simulink model "Deepanshu_GWO"  (R2021a)
settings: Solver=VariableStepAuto  StartTime=0.0  StopTime=20  FixedStep=1e-6  RelTol=1e-3
InitFcn:
  | global vv;
libraries: spsSeriesRLCBranchLib x9, spsDiodeLib x4, spsPVArrayLib x3, spsVoltageMeasurementLib x3, spsCurrentMeasurementLib x2, spsDCVoltageSourceLib x1, spsMosfetLib x1, eePwmGenerator x1, spspowerguiLib x1
settings Model: Creator=dfcpstage17  LastModifiedBy=sanr14
settings DebuggingCC: UnconnectedInputMsg=none  UnconnectedOutputMsg=none  UnconnectedLineMsg=none
settings RTWCC: DLArmComputeVersion=20.02.1

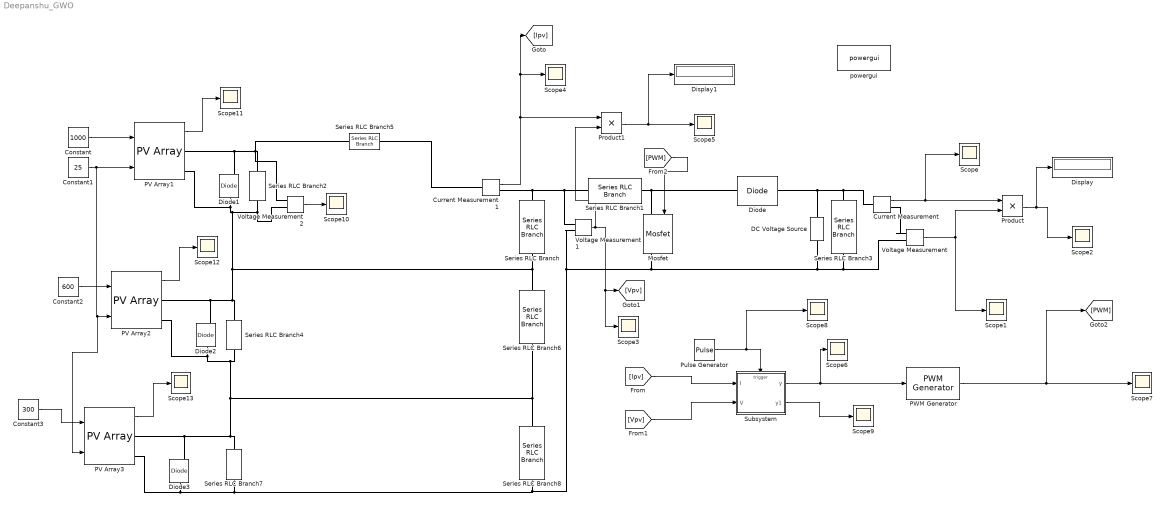
== system Deepanshu_GWO ==
  Constant : Constant  Value=1000
  Constant1 : Constant  Value=25
  Constant2 : Constant  Value=600
  Constant3 : Constant  Value=300
  Current Measurement : spsCurrentMeasurementLib/Current Measurement  PhasorSimulation=off  OutputType=Complex  PSBequivalent=0
  Current Measurement1 : spsCurrentMeasurementLib/Current Measurement  PhasorSimulation=off  OutputType=Complex  PSBequivalent=0
  DC Voltage Source : spsDCVoltageSourceLib/DC Voltage Source  Amplitude=80  Measurements=None
  Diode : spsDiodeLib/Diode  Ron=0.001  Lon=0  Vf=0.8  IC=0  UseSnubber=0  Rs=500  Cs=250e-9  Measurements=off
  Diode1 : spsDiodeLib/Diode  Ron=0.001  Lon=0  Vf=0.8  IC=0  UseSnubber=0  Rs=inf  Cs=inf  Measurements=on
  Diode2 : spsDiodeLib/Diode  Ron=0.001  Lon=0  Vf=0.8  IC=0  UseSnubber=0  Rs=inf  Cs=inf  Measurements=on
  Diode3 : spsDiodeLib/Diode  Ron=0.001  Lon=0  Vf=0.8  IC=0  UseSnubber=0  Rs=inf  Cs=inf  Measurements=on
  Display : Display
  Display1 : Display
  Mosfet : spsMosfetLib/Mosfet  Ron=0.1  Lon=0  Rd=0.01  Vfd=0  IC=0  Rs=1e5  Cs=inf  Measurements=on
  PV Array1 : spsPVArrayLib/PV Array  Npar=1  Nser=1  PlotType=array @ 1000 W/m2 & specified temperatures  S_vec="[ 1000  500  100 ]"  Temp_C_vec="[ 45 25  ]"  ModuleName=User-defined  PlotWhenSelected=off  Pm=86.996  Ncell=36  Voc=21  Isc=5.17  Vm=18.2  Im=4.78  beta_Voc_pc=-0.3616  alpha_Isc_pc=0.041509  beta_Voc=-0.075936  alpha_Isc=0.002146  IL=5.1832  I0=1.7804e-10  nI=0.94398  Rsh=97.5456  Rs=0.017583  RobustModel=off  RobustCellTemperature=313.3991  BAL=on  Tc=1e-6  Tfilter=5e-5
  PV Array2 : spsPVArrayLib/PV Array  Npar=1  Nser=1  PlotType=array @ 1000 W/m2 & specified temperatures  S_vec="[ 1000  500  100 ]"  Temp_C_vec="[ 45 25  ]"  ModuleName=User-defined  PlotWhenSelected=off  Pm=86.996  Ncell=36  Voc=21  Isc=5.17  Vm=18.2  Im=4.78  beta_Voc_pc=-0.3616  alpha_Isc_pc=0.041509  beta_Voc=-0.075936  alpha_Isc=0.002146  IL=5.1832  I0=1.7804e-10  nI=0.94398  Rsh=97.5456  Rs=0.017583  RobustModel=off  RobustCellTemperature=313.3991  BAL=on  Tc=1e-6  Tfilter=5e-5
  PV Array3 : spsPVArrayLib/PV Array  Npar=1  Nser=1  PlotType=array @ 1000 W/m2 & specified temperatures  S_vec="[ 1000  500  100 ]"  Temp_C_vec="[ 45 25  ]"  ModuleName=User-defined  PlotWhenSelected=off  Pm=86.996  Ncell=36  Voc=21  Isc=5.17  Vm=18.2  Im=4.78  beta_Voc_pc=-0.3616  alpha_Isc_pc=0.041509  beta_Voc=-0.075936  alpha_Isc=0.002146  IL=5.1832  I0=1.7804e-10  nI=0.94398  Rsh=97.5456  Rs=0.017583  RobustModel=off  RobustCellTemperature=313.3991  BAL=on  Tc=1e-6  Tfilter=5e-5
  PWM Generator : eePwmGenerator/PWM Generator  CarrCount=Up  Tper=0.0001  Ts=5e-6
  Product : Product
  Product1 : Product
  Pulse Generator : DiscretePulseGenerator  PulseType=Time based  Period=0.2  PulseWidth=30  PhaseDelay=1e-6
  Scope{,1..13} (14 alike) : Scope
  Series RLC Branch : spsSeriesRLCBranchLib/Series RLC Branch  LConnTagsString=__new0  RConnTagsString=__new0  BranchType=C  Resistance=1  Inductance=1e-3  SetiL0=off  InitialCurrent=0  Capacitance=1000e-6  Setx0=off  InitialVoltage=0  Measurements=None
  Series RLC Branch1 : spsSeriesRLCBranchLib/Series RLC Branch  LConnTagsString=__new0  RConnTagsString=__new0  BranchType=L  Resistance=1  Inductance=1e-3  SetiL0=off  InitialCurrent=0  Capacitance=1e-6  Setx0=off  InitialVoltage=0  Measurements=None
  Series RLC Branch{2..4,7} (4 alike) : spsSeriesRLCBranchLib/Series RLC Branch  LConnTagsString=__new0  RConnTagsString=__new0  BranchType=R  Resistance=100  Inductance=1e-3  SetiL0=off  InitialCurrent=0  Capacitance=1e-6  Setx0=off  InitialVoltage=0  Measurements=None
  Series RLC Branch5 : spsSeriesRLCBranchLib/Series RLC Branch  LConnTagsString=__new0  RConnTagsString=__new0  BranchType=R  Resistance=0.01  Inductance=1e-3  SetiL0=off  InitialCurrent=0  Capacitance=1e-6  Setx0=off  InitialVoltage=0  Measurements=None
  Series RLC Branch6 : spsSeriesRLCBranchLib/Series RLC Branch  LConnTagsString=__new0  RConnTagsString=__new0  BranchType=C  Resistance=1  Inductance=1e-3  SetiL0=off  InitialCurrent=0  Capacitance=1000e-6  Setx0=off  InitialVoltage=0  Measurements=None
  Series RLC Branch8 : spsSeriesRLCBranchLib/Series RLC Branch  LConnTagsString=__new0  RConnTagsString=__new0  BranchType=C  Resistance=1  Inductance=1e-3  SetiL0=off  InitialCurrent=0  Capacitance=1000e-6  Setx0=off  InitialVoltage=0  Measurements=None
  Subsystem : Subsystem
  Voltage Measurement : spsVoltageMeasurementLib/Voltage Measurement  PhasorSimulation=off  OutputType=Complex  PSBequivalent=0
  Voltage Measurement1 : spsVoltageMeasurementLib/Voltage Measurement  PhasorSimulation=off  OutputType=Complex  PSBequivalent=0
  Voltage Measurement2 : spsVoltageMeasurementLib/Voltage Measurement  PhasorSimulation=off  OutputType=Complex  PSBequivalent=0
  powergui : spspowerguiLib/powergui  Priority=1  SimulationMode=Discrete  SampleTime=1e-6  frequency=60  Iterations=50  frequencyindice=0  Pbase=100e6  ErrMax=1e-4  UnitsV=kV  UnitsW=MW  buscounter=0  FunctionMessages=off  echomessages=off  EnableUseOfTLC=off  CurrentSourceSwitches=off  DisableSnubberDevices=off  DisableRonSwitches=off  DisableVfSwitches=off  DisplayEquations=off  AutomaticDiscreteSolvers=off  SolverType=Tustin/Backward Euler (TBE)  Interpol=off  ExternalGateDelay=off  methode=off  Ts=100  x0status=blocks  SPID=on  SwTol=0  HookPort=off  NonlinearTolerance=1e-4  nMaxIteration=100  ContinueOnMaxIteration=off  RestoreLinks=warning  ResistiveCurrentMeasurement=off  Frange=[0:2:500]  Ylog=off  Xlog=on  ShowGrid=off  save=off  variable=ZData  structure=0  ZoomFFT=off  StartTime=0.0  cycles=1  DisplayStyle=1  fundamental=60  FreqAxis=off  MaxFrequency=1000  frequencyindicesteady=1  RmsSteady=1  display=off
  wires:
  Current Measurement/1 -> Scope/1, Product/1
  Voltage Measurement/1 -> Product/2, Scope1/1
  Product/1 -> Display/1, Scope2/1
  Voltage Measurement1/1 -> Product1/2, [Vpv], Scope3/1
  Current Measurement1/1 -> Product1/1, [Ipv], Scope4/1
  Product1/1 -> Display1/1, Scope5/1
  [Ipv] -> Subsystem/1(I)
  [Vpv] -> Subsystem/2(V)
  Pulse Generator/1 -> Scope8/1, Subsystem/Trigger
  PWM Generator/1 -> Scope7/1, [PWM]
  [PWM] -> Mosfet/1
  Subsystem/1(y) -> Scope6/1, PWM Generator/1
  Constant/1 -> PV Array1/1
  Constant1/1 -> PV Array3/2, PV Array2/2, PV Array1/2
  Subsystem/2(y1) -> Scope9/1
  Voltage Measurement2/1 -> Scope10/1
  PV Array1/1 -> Scope11/1
  PV Array2/1 -> Scope12/1
  Constant2/1 -> PV Array2/1
  PV Array3/1 -> Scope13/1
  Constant3/1 -> PV Array3/1
  connections:
  Series RLC Branch1/LConn1 -- Voltage Measurement1/LConn1 -- Current Measurement1/RConn1 -- Series RLC Branch/LConn1
  Mosfet/LConn1 -- Diode/LConn1 -- Series RLC Branch1/RConn1
  Diode/RConn1 -- DC Voltage Source/RConn1 -- Series RLC Branch3/LConn1 -- Current Measurement/LConn1
  Voltage Measurement/LConn1 -- Current Measurement/RConn1
  PV Array1/RConn1 -- Diode1/RConn1 -- Series RLC Branch5/RConn1 -- Voltage Measurement2/LConn1 -- Series RLC Branch2/LConn1
  Series RLC Branch5/LConn1 -- Current Measurement1/LConn1
  Series RLC Branch6/LConn1 -- Series RLC Branch4/LConn1 -- Diode2/RConn1 -- PV Array2/RConn1 -- PV Array1/RConn2 -- Diode1/LConn1 -- Voltage Measurement2/LConn2 -- Series RLC Branch2/RConn1 -- Series RLC Branch/RConn1
  Voltage Measurement1/LConn2 -- PV Array3/RConn2 -- Diode3/LConn1 -- Series RLC Branch7/RConn1 -- Series RLC Branch8/RConn1 -- DC Voltage Source/LConn1 -- Voltage Measurement/LConn2 -- Series RLC Branch3/RConn1 -- Mosfet/RConn1
  PV Array2/RConn2 -- Series RLC Branch6/RConn1 -- Series RLC Branch8/LConn1 -- Diode3/RConn1 -- PV Array3/RConn1 -- Series RLC Branch7/LConn1 -- Series RLC Branch4/RConn1 -- Diode2/LConn1

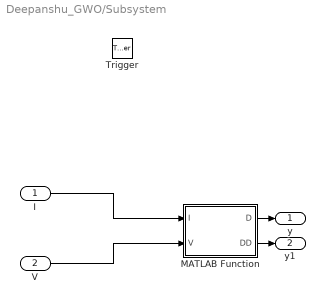
== system Deepanshu_GWO/Subsystem ==
  I : Inport
  V : Inport  Port=2
  Trigger : TriggerPort  VariantControl=(inherit)  PortDimensions=1
  MATLAB Function : MATLAB Function  TreatAsAtomicUnit=on
  y : Outport
  y1 : Outport  Port=2
  wires:
  V/1 -> MATLAB Function/2(V)
  I/1 -> MATLAB Function/1(I)
  MATLAB Function/1(D) -> y/1
  MATLAB Function/2(DD) -> y1/1

== matlab function Deepanshu_GWO/Subsystem/MATLAB Function ==
  data: I input; D output; V input; DD output
function [D, DD] = d(I,V)

    % Parameters
    N = 10;           % Number of grey wolves (search agents)

    persistent Ini_count;
    if (isempty(Ini_count))
        Ini_count = 0;
    end
    Ini_count = Ini_count + 1;
    if(Ini_count > 20)
        Ini_count = 11;
    end

    persistent Ini_done;
    if (isempty(Ini_done))
        Ini_done = 0;
     end
%========================================================================== 
    persistent j;
    if (isempty(j))
        j = 0;
     end
%========================================================================== 
    persistent BestPower;
    if (isempty(BestPower))
        BestPower = 0;
    end

    persistent StoppingCriteria;
    if (isempty(StoppingCriteria))
        StoppingCriteria = 0;
    end

    persistent bestIdx;
    if (isempty(bestIdx))
        bestIdx = 1;
    end
    
    persistent X ;    % Initial positions of the search agents
    if (isempty(X)) 
        X = [0.2 0.25 0.3 0.4 0.45 0.5 0.6 0.65 0.7 0.8];
    end

    persistent X_new ;  % New positions of the search agents
    if (isempty(X_new)) 
        X_new = zeros(1,N);
    end

    persistent X_best ; % Best solution found so far
    if (isempty(X_best)) 
        X_best = 0;
    end

    persistent X_best_global ; % Best solution found so far
    if (isempty(X_best_global)) 
        X_best_global = 0;
    end

    persistent alphaPos;
    if (isempty(alphaPos)) 
        alphaPos = 0;
    end

    persistent betaPos;
    if (isempty(betaPos))
        betaPos = 0;
    end

    persistent deltaPos;
    if (isempty(deltaPos))
        deltaPos = 0;
    end

    persistent alphaScore;
    if (isempty(alphaScore)) 
        alphaScore = 0;
    end

    persistent betaScore;
    if (isempty(betaScore))
        betaScore = 0;
    end

    persistent deltaScore;
    if (isempty(deltaScore))
        deltaScore= 0;
    end

    persistent Fitness;
    if(isempty(Fitness))
    Fitness= [0 0 0 0 0 0 0 0 0 0];    % Initialize fitness array for each iteration
    end

    persistent i;
    if(isempty(i))
        i=0;
    end
 
    if(i>1.99)
        i=0;
    end

    persistent p;
    if(isempty(p))
        p=1;
    end
%==========================================================================
%      
%     if j == 10
% 
%         if (abs(BestPower - Fitness(bestIdx)) < 2 )
%             StoppingCriteria = 1 ;
%         else 
%             StoppingCriteria = 0 ;
%         end
% 
%         if Fitness(bestIdx) > BestPower
%             X_best_global = X_best;
%             BestPower = Fitness(bestIdx);
%         end
% 
%     end
% 






%   if(StoppingCriteria==0)
%==========================================================================

%%%%%%%%%%%%%%%%%%%%%%%%%%%%%%%%%%%%%%%%%%%%%%%%%%%%%%%%%%%%%%%%%%%%%%%%%%%%%%%%%%%%%%%%%%%%%%%%%%%%%%%%%%%%%%%%%%%%%%%%%%%%%%%%%%%%%%%%%%%%%%%%%%%
    D = X(1);
if(Ini_count < 11)
    D = X(Ini_count);
    if(Ini_count > 1)
        Fitness(Ini_count-1) = V * I;
    end
    if(Ini_count == 10)
        Ini_done = 1;
    end
end

if(Ini_count >= 11)
    if(Ini_done == 1)
        Fitness(Ini_count-1) = V * I;
        Ini_done = 0;
    end
    %%%%%%%%%%%%%%%%%%%%%%%%%%%%%%%%%%%%%%%%%%%%%%%%%%%%%%%%%%%%%%%%%%%%%%%%%%%%%%%%%%%%%%%%%%%% Codes
    for j=1:10
        if(Fitness(j) > alphaScore)
            alphaScore = Fitness(j);
            alphaPos = X(j);
        end
        if((Fitness(j) > betaScore) && (Fitness(j) < alphaScore))
            betaScore = Fitness(j);
            betaPos = X(j);
        end
        if((Fitness(j) > deltaScore) && (Fitness(j) < betaScore))
            deltaScore = Fitness(j);
            deltaPos = X(j);
        end
    end

    %C1 = 1.7;
        a = 1.5;
        r1 = 0.4 + 0.2 * rand(1);  % Nombre aléatoire pour mise à jour
        r2 = 0.4 + 0.2 * rand(1);  % Nombre aléatoire pour mise à jour
        A1 = 2 * a * r1 - a;  % Facteur d'actualisation
        C1 = 2 * r2;  % Coefficient de mise à jour
    Dalpha = (C1 * alphaPos - X(Ini_count - 10));%abs(C1 * alphaPos - X(Ini_count - 10)); 
    %A1 = 0.2;
    X1= alphaPos - A1* Dalpha;

    %C2 = 0.2;
        r1 = 0.4 + 0.2 * rand(1);  % Nombre aléatoire pour mise à jour
        r2 = 0.4 + 0.2 * rand(1);  % Nombre aléatoire pour mise à jour
        A2 = 2 * a * r1 - a;  % Facteur d'actualisation
        C2 = 2 * r2;  % Coefficient de mise à jour
    Dbeta = (C2 * betaPos - X(Ini_count - 10));%abs(C2 * betaPos - X(Ini_count - 10)); 
    %A2 = 0.2;
    X2= betaPos - A2 * Dbeta;

    %C3 = 0.05;
        r1 = 0.4 + 0.2 * rand(1);  % Nombre aléatoire pour mise à jour
        r2 = 0.4 + 0.2 * rand(1);  % Nombre aléatoire pour mise à jour
        A3 = 2 * a * r1 - a;  % Facteur d'actualisation
        C3 = 2 * r2;  % Coefficient de mise à jour
    Ddelta = (C3 * deltaPos - X(Ini_count - 10));%abs(C3 * deltaPos - X(Ini_count - 10));  
    %A3 = 0.2;
    X3= deltaPos - A3 * Ddelta;

    X(Ini_count - 10) = (X1 + X2 + X3) / 3;
    D = X(Ini_count - 10);

    if (Ini_count > 11)
        Fitness(Ini_count-11) = V * I;
    end
    if ((Ini_count == 11) && (Ini_done == 0))
        Fitness(10) = V * I;
    end
    %%%%%%%%%%%%%%%%%%%%%%%%%%%%%%%%%%%%%%%%%%%%%%%%%%%%%%%%%%%%%%%%%%%%%%%%%%%%%%%%%%%%%%%%%%%% End_Codes
end
%%%%%%%%%%%%%%%%%%%%%%%%%%%%%%%%%%%%%%%%%%%%%%%%%%%%%%%%%%%%%%%%%%%%%%%%%%%%%%%%%%%%%%%%%%%%%%%%%%%%%%%%%%%%%%%%%%%%%%%%%%%%%%%%%%%%%%%%%%%%%%%%%%%





%     % Generate 10 different powers for each wolf
%    
%     if j == 0
%         D = X(j+1);
% 
%     elseif j <= 10
%         % Calculate power
%         Pmeas = I * V;
%         % Store power in fitness
%         Fitness(j) = Pmeas;  % Fitness for each wolf       
% 
%         % Find the best solution (maximum power output)
%         [~, bestIdx] = max(Fitness);
%         X_best = X(bestIdx);
%         %fprintf('best duty = %1.0f',X_best);
% 
%          
%         if alphaScore < Fitness(bestIdx)               
%            alphaScore=Fitness(bestIdx);
%            alphaPos=X_best;
%         end
%     
%         if (alphaScore> Fitness(j)) && (betaScore < Fitness(j))
%            betaScore=Fitness(j);
%            betaPos=X(j);
%         end
%     
%         if (betaScore> Fitness(j)) && (deltaScore < Fitness(j))
%            deltaScore = Fitness(j);
%            deltaPos = X(j);
%         end
%     end
% 
%    
% 
%     if (0 < j) && (j < 10)
%         D = X(j+1);
% 
%     else
%         D = X_best;
%   
%     end
% %==========================================================================
% 
%     % Update the position of current wolf
% 
%     if j > 0
%         a = 2-i;  % alteration factor
% 
%         r1 = rand(1); %0.3 + 0.5 * rand(1);  % Nombre aléatoire pour mise à jour
%         r2 = rand(1); % 0.3 + 0.5 * rand(1);  % Nombre aléatoire pour mise à jour
%         A1 = 2 * a * r1 - a;  % Facteur d'actualisation
%         C1 = 2 * r2;  % Coefficient de mise à jour
%         Dalpha = abs(C1 * alphaPos - X(j));  
%         A1 = 0.2;
%         X1= alphaPos - A1* Dalpha; 
% 
%         %fprintf('X1 = %1.0f',X1);
%         % r1 = rand(1); % 0.3 + 0.5 * rand(1);  % Nombre aléatoire pour mise à jour
%         % r2 = rand(1); % 0.3 + 0.5 * rand(1);  % Nombre aléatoire pour mise à jour
%         A2 = 2 * a * r1 - a;  % Facteur d'actualisation
%         C2 = 2 * r2;  % Coefficient de mise à jour
%         Dbeta = abs(C2 * betaPos - X(j));  
%         A2 = 0.2;
%         X2= betaPos - A2 * Dbeta; 
%         
%         % r1 = rand(1); % 0.3 + 0.5 * rand(1);  % Nombre aléatoire pour mise à jour
%         % r2 = rand(1); % 0.3 + 0.5 * rand(1);  % Nombre aléatoire pour mise à jour
%         A3 = 2 * a * r1 - a;  % Facteur d'actualisation
%         C3 = 2 * r2;  % Coefficient de mise à jour
%         Ddelta = abs(C3 * deltaPos - X(j)); 
%         A3 = 0.2;
%         X3= deltaPos - A3 * Ddelta; 
% 
%         % Update the positions of the search agent
%         X(j) = (X1 + X2 + X3) / 3;
% 
%         %fprintf('X %1.0f = %1.0f',j, X(j) );
% 
%         if(X(j)>0.9)
%             X(j) = 0.9;
%         end
%         if(X(j)<0.1)
%             X(j) = 0.1;
%         end
% 
%         i=i+0.03;
%    
%     end
% %   else 
% 
% 
%     
%         
% 
% %==========================================================================
% 
%     DD = X; 
%     DDD = j;
% 
%     j = j + 1;
% 
% 
%     % fprintf('Duty Cycle = %1.0f',max(X_new));
%     % fprintf('Duty Cycle = %1.0f',min(X_new));
%     %fprintf('Fitness = %1.0f',Fitness(1));
fprintf('iteration = %1.0f',Ini_count);
fprintf('Power = %1.0f',Fitness(1));
fprintf('Power = %1.0f',Fitness(2));
fprintf('Power = %1.0f',Fitness(3));
fprintf('Power = %1.0f',Fitness(4));
fprintf('Power = %1.0f',Fitness(5));
fprintf('Power = %1.0f',Fitness(6));
fprintf('Power = %1.0f',Fitness(7));
fprintf('Power = %1.0f',Fitness(8));
fprintf('Power = %1.0f',Fitness(9));
fprintf('Power = %1.0f',Fitness(10));
fprintf('Alp = %1.2f',alphaPos);
fprintf('ALp_Power = %1.2f',alphaScore);
fprintf('Bet = %1.2f',betaPos);
fprintf('Bet_Power = %1.2f',betaScore);
fprintf('Del = %1.2f',deltaPos);
fprintf('Del_Power = %1.2f',deltaScore);
DD = 0;
end
